simulink model "Portefolio_2_2"  (Simulink 7.5)
settings: Solver=ode45  StartTime=0.0  StopTime=10  MaxStep=0.01  RelTol=1e-3
values from neighbouring files (symbols this model uses):
  A = 1/(k1^2 - k4^2)*[k3*k4 k1*k3; k1*k3 k3*k4]    [portfolie_2_better.m]
  b = 0.26    [portfolie_2_better.m]    (also in portfolie_2_lol.m)
  B = 1/(k1^2 - k4^2)*[(-k2)*k4 (-k1)*k2; (-k1)*k2 (-k2)*k4]    [portfolie_2_better.m]
  C = [1 0; 0 1]    [portfolie_2_better.m]
  K = [35 10; 10 35]    [portfolie_2_better.m]
  L = 4 * K    [portfolie_2_better.m]
  r = 0.1    [portfolie_2_better.m]    (also in portfolie_2_lol.m)
  sys = ss(A,B,C,D)    [portfolie_2_better.m]    (also in portfolie_2_lol.m = canon(G,'modal'))
libraries: simulink x3
settings Model: Creator=Jeppe Pedersen  LastModifiedBy=Jeppe Pedersen

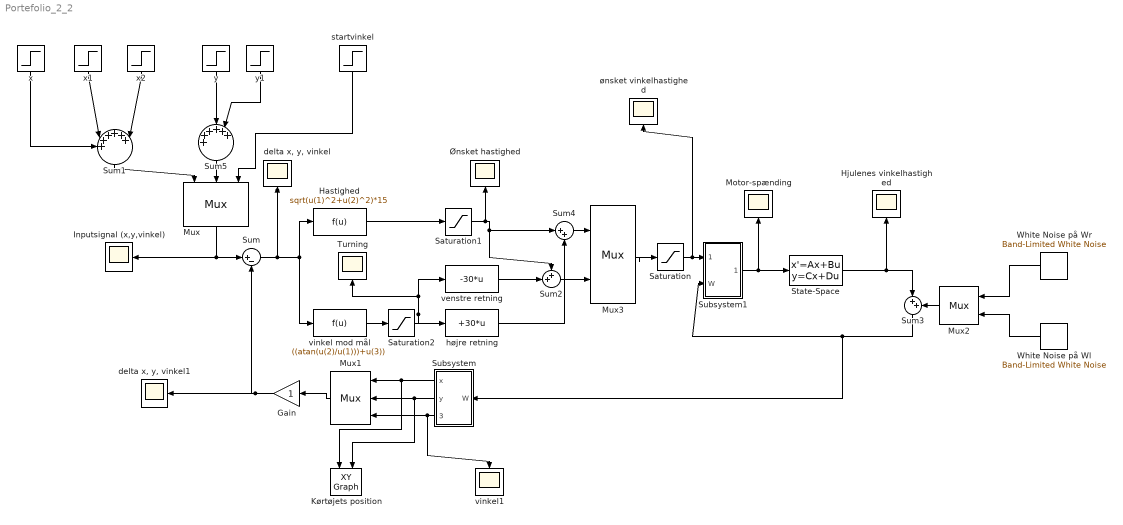
== system Portefolio_2_2 ==
  Gain : Gain  ParameterDataType=fixdt(1, 16)  ParameterScaling=2^0  OutDataType=fixdt(1, 16)  OutScaling=2^0
  Hastighed : Fcn  Expr=sqrt(u(1)^2+u(2)^2)*15
  Hjulenes vinkelhastighed : Scope
  Inputsignal (x,y,vinkel) : Scope
  Kørtøjets position : simulink/Sinks/XY Graph  SystemSampleTime=-1  xmin=-0.2  xmax=2  ymin=-0.2  ymax=2  st=-1
  Motor-spænding : Scope
      settings: SaveName=ScopeData2
  Mux : Mux  Inputs=3
      settings: DisplayOption=signals
  Mux1 : Mux  Inputs=3
      settings: DisplayOption=signals
  Mux2 : Mux  Inputs=2
      settings: DisplayOption=signals
  Mux3 : Mux  Inputs=2
      settings: DisplayOption=signals
  Saturation : Saturate  UpperLimit=6  LowerLimit=-6  OutDataType=fixdt(1, 16)  OutScaling=2^0
  Saturation1 : Saturate  UpperLimit=6  LowerLimit=-6  OutDataType=fixdt(1, 16)  OutScaling=2^0
  Saturation2 : Saturate  UpperLimit=pi/2  LowerLimit=-pi/2  OutDataType=fixdt(1, 16)  OutScaling=2^0
  State-Space : StateSpace  A=sys.A  B=sys.B  C=sys.C  D=sys.D
  Subsystem : Subsystem
  Subsystem1 : Subsystem
  Sum : Sum  Inputs=|+-  OutDataType=fixdt(1, 16)  OutScaling=2^0
  Sum1 : Sum  Inputs=++++++|  OutDataType=fixdt(1, 16)  OutScaling=2^0
  Sum2 : Sum  Inputs=++|  OutDataType=fixdt(1, 16)  OutScaling=2^0
  Sum3 : Sum  Inputs=|++  OutDataType=fixdt(1, 16)  OutScaling=2^0
  Sum4 : Sum  Inputs=|++  OutDataType=fixdt(1, 16)  OutScaling=2^0
  Sum5 : Sum  Inputs=++++++|  OutDataType=fixdt(1, 16)  OutScaling=2^0
  Turning : Scope
      settings: SaveName=ScopeData6
  White Noise på Wl : simulink/Sources/Band-Limited White Noise  SystemSampleTime=-1  Cov=0  Ts=0.01  seed=[27741]
  White Noise på Wr : simulink/Sources/Band-Limited White Noise  SystemSampleTime=-1  Cov=0  Ts=0.01  seed=[23341]
  "delta x, y, vinkel" : Scope
      settings: SaveName=ScopeData3
  "delta x, y, vinkel1" : Scope
      settings: SaveName=ScopeData7
  højre retning : Fcn  Expr=+30*u
  startvinkel : Step  Time=0  After=0  SampleTime=0
  venstre retning : Fcn  Expr=-30*u
  vinkel mod mål : Fcn  Expr=((atan(u(2)/u(1)))+u(3))
  vinkel1 : Scope
      settings: SaveName=ScopeData4
  x : Step  Before=0.01  SampleTime=0
  x1 : Step  Time=4  After=sqrt(2)/2  SampleTime=0
  x2 : Step  Time=3  After=0  SampleTime=0
  y : Step  Time=4  After=sqrt(2)/2  SampleTime=0
  y1 : Step  Time=0  After=0  SampleTime=0
  Ønsket hastighed : Scope
      settings: SaveName=ScopeData8
  ønsket vinkelhastighed : Scope
      settings: SaveName=ScopeData5
  wires:
  State-Space/1 -> Hjulenes vinkelhastighed/1, Sum3/1
  Mux/1 -> Inputsignal (x,y,vinkel)/1, Sum/1
  Sum3/1 -> Subsystem/1(W), Subsystem1/2(W)
  Subsystem1/1(u [V]) -> State-Space/1, Motor-spænding/1
  Mux1/1 -> Gain/1
  Subsystem/1(x) -> Mux1/1, Kørtøjets position/1
  Subsystem/2(y) -> Mux1/2, Kørtøjets position/2
  Subsystem/3(vinkel) -> vinkel1/1, Mux1/3
  Gain/1 -> Sum/2, "delta x, y, vinkel1"/1
  White Noise på Wr/1 -> Mux2/1
  White Noise på Wl/1 -> Mux2/2
  Mux2/1 -> Sum3/2
  x1/1 -> Sum1/2
  x/1 -> Sum1/1
  Sum/1 -> "delta x, y, vinkel"/1, Hastighed/1, vinkel mod mål/1
  Sum1/1 -> Mux/1
  Saturation/1 -> Subsystem1/1(Wd), ønsket vinkelhastighed/1
  startvinkel/1 -> Mux/3
  Mux3/1 -> Saturation/1
  Saturation1/1 -> Sum2/1, Sum4/1, Ønsket hastighed/1
  Sum4/1 -> Mux3/1
  Sum2/1 -> Mux3/2
  venstre retning/1 -> Sum2/2
  højre retning/1 -> Sum4/2
  x2/1 -> Sum1/6
  y/1 -> Sum5/4
  Sum5/1 -> Mux/2
  y1/1 -> Sum5/5
  vinkel mod mål/1 -> Saturation2/1
  Saturation2/1 -> Turning/1, venstre retning/1, højre retning/1
  Hastighed/1 -> Saturation1/1

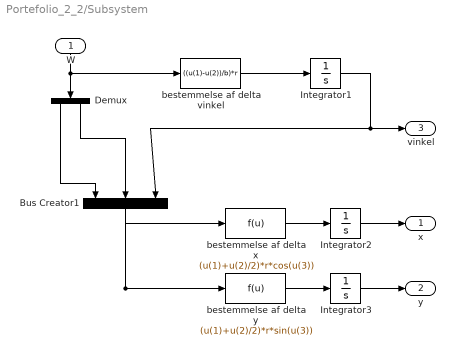
== system Portefolio_2_2/Subsystem ==
  W : Inport
  Bus Creator1 : BusCreator  Inputs=3
  Demux : Demux  Outputs=2
  Integrator1 : Integrator
  Integrator2 : Integrator
  Integrator3 : Integrator
  bestemmelse af delta vinkel : Fcn  Expr=((u(1)-u(2))/b)*r
  bestemmelse af delta x : Fcn  Expr=(u(1)+u(2)/2)*r*cos(u(3))
  bestemmelse af delta y : Fcn  Expr=(u(1)+u(2)/2)*r*sin(u(3))
  x : Outport
  y : Outport  Port=2
  vinkel : Outport  Port=3
  wires:
  Demux/1 -> Bus Creator1/1
  Demux/2 -> Bus Creator1/2
  Bus Creator1/1 -> bestemmelse af delta x/1, bestemmelse af delta y/1
  Integrator3/1 -> y/1
  bestemmelse af delta y/1 -> Integrator3/1
  Integrator2/1 -> x/1
  bestemmelse af delta x/1 -> Integrator2/1
  Integrator1/1 -> Bus Creator1/3, vinkel/1
  bestemmelse af delta vinkel/1 -> Integrator1/1
  W/1 -> Demux/1, bestemmelse af delta vinkel/1

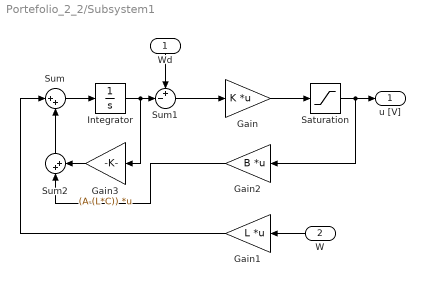
== system Portefolio_2_2/Subsystem1 ==
  Wd : Inport
  W : Inport  Port=2
  Gain : Gain  Gain=K  Multiplication=Matrix(K*u)  ParameterDataType=fixdt(1, 16)  ParameterScaling=2^0  OutDataType=fixdt(1, 16)  OutScaling=2^0
  Gain1 : Gain  Gain=L  Multiplication=Matrix(K*u)  ParameterDataType=fixdt(1, 16)  ParameterScaling=2^0  OutDataType=fixdt(1, 16)  OutScaling=2^0
  Gain2 : Gain  Gain=B  Multiplication=Matrix(K*u)  ParameterDataType=fixdt(1, 16)  ParameterScaling=2^0  OutDataType=fixdt(1, 16)  OutScaling=2^0
  Gain3 : Gain  Gain=(A-(L*C))  Multiplication=Matrix(K*u)  ParameterDataType=fixdt(1, 16)  ParameterScaling=2^0  OutDataType=fixdt(1, 16)  OutScaling=2^0
  Integrator : Integrator
  Saturation : Saturate  UpperLimit=12  LowerLimit=-12  OutDataType=fixdt(1, 16)  OutScaling=2^0
  Sum : Sum  Inputs=|++  OutDataType=fixdt(1, 16)  OutScaling=2^0
  Sum1 : Sum  Inputs=+-|  OutDataType=fixdt(1, 16)  OutScaling=2^0  InputSameDT=on
  Sum2 : Sum  Inputs=|++  OutDataType=fixdt(1, 16)  OutScaling=2^0
  u [V] : Outport
  wires:
  Gain/1 -> Saturation/1
  Gain1/1 -> Sum/1
  Sum/1 -> Integrator/1
  Integrator/1 -> Sum1/2, Gain3/1
  Sum1/1 -> Gain/1
  Gain3/1 -> Sum2/2
  Gain2/1 -> Sum2/1
  Sum2/1 -> Sum/2
  Saturation/1 -> Gain2/1, u [V]/1
  Wd/1 -> Sum1/1
  W/1 -> Gain1/1
